simulink model "MRI_2D_FFT"  (R2020a)
settings: Solver=VariableStepAuto  StartTime=0.0  StopTime=256*256*11+2000  RelTol=1e-3  EnableMultiTasking=on
PreLoadFcn:
  | MRI_2D_FFT_PreloadFcn
undefined symbols (not defined in the file): col_in, col_out, corner_turn_memory_depth, row_in, xlFrameDisplay
libraries: xbsIndex_r4 x83, dspswit3 x2, dspsrcs4 x2, xbsCopyrightNotice_r4 x1, simulink x1
settings Model: Creator=dahlawat  LastModifiedBy=viswanad
settings DataIOCC: LimitDataPoints=on  ReturnWorkspaceOutputs=off
settings OptimizationCC: LifeSpan=inf
settings DebuggingCC: AllowSymbolicDim=off  SFUnexpectedBacktrackingDiag=warning  SFNoUnconditionalDefaultTransitionDiag=warning  SFExecutionAtInitializationDiag=none  ArithmeticOperatorsInVariantConditions=warning
settings ModelReferenceCC: PropagateSignalLabelsOutOfModel=off
settings SFSimCC: SimUseLocalCustomCode=off  CustomCodeUndefinedFunction=UseInterfaceOnly
settings RTWCC: RTWUseLocalCustomCode=off
settings CodeAppCC: StateflowObjectComments=on
settings GRTTargetCC: TargetLangStandard=C89/C90 (ANSI)
settings ConfigComp: CovMetricSettings=dw  CovSaveCumulativeToWorkspaceVar=on  CovSaveSingleToWorkspaceVar=on  CovExternalEMLEnable=off

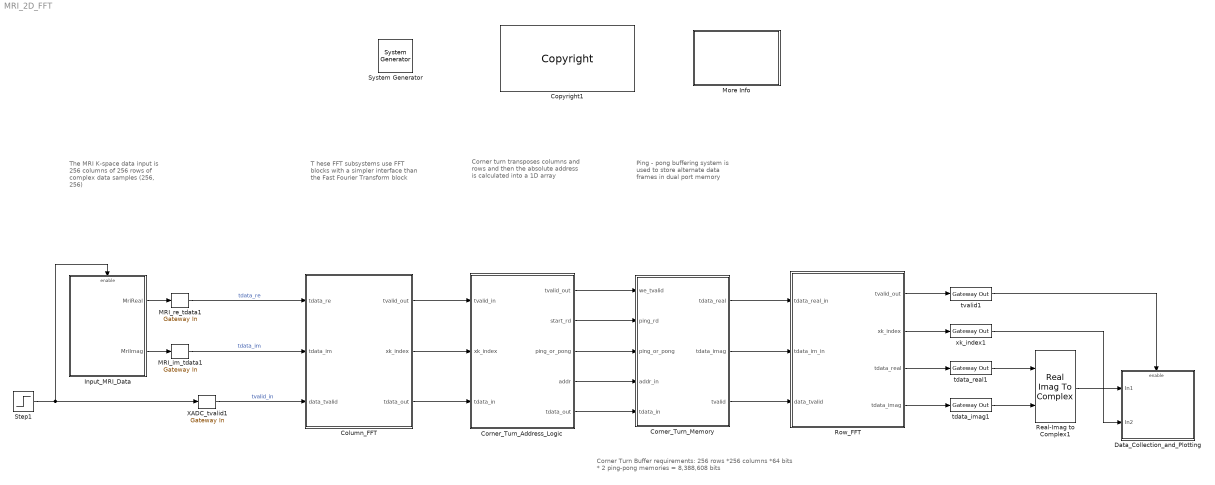
== system MRI_2D_FFT ==
  note: T hese FFT subsystems use FFT blocks with a simpler interface than the Fast Fourier Transform block
  note: Corner Turn Buffer requirements: 256 rows *256 columns *64 bits * 2 ping-pong memories = 8,388,608 bits
  note: The MRI K-space data input is 256 columns of 256 rows of complex data samples
      | (256, 256)
  note: Corner turn transposes columns and rows and then the absolute address is calculated into a 1D array
  note: Ping - pong buffering system is used to store alternate data frames in dual port memory
  " System Generator" : xbsIndex_r4/ System Generator  Tag=genX  xilinxfamily=zynquplus  part=xczu7ev  speed=-2-e  package=ffvc1156  synthesis_tool=Vivado  clock_wrapper=Clock Enables  directory=./netlist  proj_type=Vivado  Synth_file=Vivado Synthesis Defaults  Impl_file=Vivado Implementation Defaults  testbench=on  simulink_period=1  sysclk_period=10  dcm_input_clock_period=10  incr_netlist=off  trim_vbits=Everywhere in SubSystem  dbl_ovrd=According to Block Masks  core_generation=According to Block Masks  run_coregen=off  deprecated_control=off  eval_field=0  block_type=sysgen
  Column_FFT : Subsystem
  Copyright1 : xbsCopyrightNotice_r4/Copyright  copyrighttext="Copyright (c) 2021  by  Xilinx, Inc. All rights reserved.<br><br>This file contains proprietary, confidential information of Xilinx, Inc., is distributed under license from Xilinx, Inc., and may be used, copied and/or disclosed only pursuant to the terms of a valid license agreement with Xilinx, Inc. Xilinx hereby grants you a license to use this file solely for design, simulation, implementation and creation of design files limited to Xilinx devices or technologies. Use with non-Xilinx devices or technologies is expressly prohibited and immediately terminates your license unless covered by a separate agreement.<br><br>Xilinx is providing this design, code, or information \"as-is\" solely for use in developing programs and solutions for Xilinx devices, with no obligation on the part of Xilinx to provide support. By providing this design, code, or information as one possible implementation of this feature, application or standard, Xilinx is making no representation that this implementation is free from any claims of infringement. You are responsible for obtaining any rights you may require for your implementation. Xilinx expressly disclaims any warranty whatsoever with respect to the adequacy of the implementation, including but not limited to any warranties or representations that this implementation is free from claims of infringement, implied warranties of merchantability or fitness for a particular purpose.<br><br>Xilinx products are not intended for use in life support appliances, devices, or systems. Use in such applications is expressly prohibited.<br><br>Any modifications that are made to the Source Code are done at the user's sole risk and will be unsupported.<br><br>This copyright and support notice must be retained as part of this text at all times. (c) Copyright 1995-2021 Xilinx, Inc. All rights reserved."  block_type=copyright
  Corner_Turn_Address_Logic : Subsystem
  Corner_Turn_Memory : Subsystem
  Data_Collection_and_Plotting : Subsystem  TreatAsAtomicUnit=on
  Input_MRI_Data : Subsystem  TreatAsAtomicUnit=on
  MRI_im_tdata1 : xbsIndex_r4/Gateway In  gui_display_data_type=Fixed-point  arith_type=Signed (2's comp)  n_bits=32  bin_pt=31  preci_type=Single  exp_width=8  frac_width=24  rows=1  columns=1  quantization=Truncate  overflow=Wrap  period=1  UseAsADC=off  ADCChannel='1'  interface=None  automatic_assignment=on  address_offset=hex2dec('00')  intf_name=''  intf_description=''  default_value=0  timing_constraint=None  locs_specified=off  LOCs={}  io_standard={}  inherit_from_input=off  hdl_port=on  XmcBlockStatus=1  maskContainerNames=group4  block_type=gatewayin  block_config=sysgen:gateway_in_config
  MRI_re_tdata1 : xbsIndex_r4/Gateway In  gui_display_data_type=Fixed-point  arith_type=Signed (2's comp)  n_bits=32  bin_pt=31  preci_type=Single  exp_width=8  frac_width=24  rows=1  columns=1  quantization=Truncate  overflow=Wrap  period=1  UseAsADC=off  ADCChannel='1'  interface=None  automatic_assignment=on  address_offset=hex2dec('00')  intf_name=''  intf_description=''  default_value=0  timing_constraint=None  locs_specified=off  LOCs={}  io_standard={}  inherit_from_input=off  hdl_port=on  XmcBlockStatus=1  maskContainerNames=group4  block_type=gatewayin  block_config=sysgen:gateway_in_config
  More Info : Subsystem
      mask Display: disp('Double click\n for\n more information.')
  Real-Imag to Complex1 : RealImagToComplex
  Row_FFT : Subsystem
  Step1 : Step  Time=64  SampleTime=1
  XADC_tvalid1 : xbsIndex_r4/Gateway In  gui_display_data_type=Boolean  arith_type=Boolean  n_bits=32  bin_pt=0  preci_type=Single  exp_width=8  frac_width=24  rows=1  columns=1  quantization="Round  (unbiased: +/- Inf)"  overflow=Saturate  period=1  UseAsADC=off  ADCChannel='1'  interface=None  automatic_assignment=on  address_offset=hex2dec('00')  intf_name=''  intf_description=''  default_value=0  timing_constraint=None  locs_specified=off  LOCs={}  io_standard={}  inherit_from_input=off  hdl_port=on  XmcBlockStatus=1  maskContainerNames=group4  block_type=gatewayin  block_config=sysgen:gateway_in_config
  tdata_imag1 : xbsIndex_r4/Gateway Out  inherit_from_input=off  hdl_port=on  rows=1  columns=1  UseAsDAC=off  DACChannel='1'  interface=None  automatic_assignment=on  address_offset=hex2dec('00')  intf_name=''  intf_description=''  timing_constraint=None  locs_specified=off  LOCs={}  io_standard={}  XmcBlockStatus=1  maskContainerNames=group4  block_type=gatewayout  block_config=sysgen:gateway_out_config
  tdata_real1 : xbsIndex_r4/Gateway Out  inherit_from_input=off  hdl_port=on  rows=1  columns=1  UseAsDAC=off  DACChannel='1'  interface=None  automatic_assignment=on  address_offset=hex2dec('00')  intf_name=''  intf_description=''  timing_constraint=None  locs_specified=off  LOCs={}  io_standard={}  XmcBlockStatus=1  maskContainerNames=group4  block_type=gatewayout  block_config=sysgen:gateway_out_config
  tvalid1 : xbsIndex_r4/Gateway Out  inherit_from_input=off  hdl_port=on  rows=1  columns=1  UseAsDAC=off  DACChannel='1'  interface=None  automatic_assignment=on  address_offset=hex2dec('00')  intf_name=''  intf_description=''  timing_constraint=None  locs_specified=off  LOCs={}  io_standard={}  XmcBlockStatus=1  maskContainerNames=group4  block_type=gatewayout  block_config=sysgen:gateway_out_config
  xk_index1 : xbsIndex_r4/Gateway Out  inherit_from_input=off  hdl_port=off  rows=1  columns=1  UseAsDAC=off  DACChannel='1'  interface=None  automatic_assignment=on  address_offset=hex2dec('00')  intf_name=''  intf_description=''  timing_constraint=None  locs_specified=off  LOCs={}  io_standard={}  XmcBlockStatus=1  maskContainerNames=group4  block_type=gatewayout  block_config=sysgen:gateway_out_config
  wires:
  Step1/1 -> Input_MRI_Data/Enable, XADC_tvalid1/1
  XADC_tvalid1/1 -> Column_FFT/3(data_tvalid)  "tvalid_in"
  Input_MRI_Data/1(MriReal) -> MRI_re_tdata1/1
  Input_MRI_Data/2(MriImag) -> MRI_im_tdata1/1
  tvalid1/1 -> Data_Collection_and_Plotting/Enable
  tdata_real1/1 -> Real-Imag to Complex1/1
  tdata_imag1/1 -> Real-Imag to Complex1/2
  Column_FFT/1(tvalid_out) -> Corner_Turn_Address_Logic/1(tvalid_in)
  Column_FFT/2(xk_index) -> Corner_Turn_Address_Logic/2(xk_index)
  Column_FFT/3(tdata_out) -> Corner_Turn_Address_Logic/3(tdata_in)
  Corner_Turn_Address_Logic/1(tvalid_out) -> Corner_Turn_Memory/1(we_tvalid)
  Corner_Turn_Address_Logic/2(start_rd) -> Corner_Turn_Memory/2(ping_rd)
  Corner_Turn_Address_Logic/3(ping_or_pong) -> Corner_Turn_Memory/3(ping_or_pong)
  Corner_Turn_Address_Logic/4(addr) -> Corner_Turn_Memory/4(addr_in)
  Corner_Turn_Address_Logic/5(tdata_out) -> Corner_Turn_Memory/5(tdata_in)
  Corner_Turn_Memory/2(tdata_imag) -> Row_FFT/2(tdata_im_in)
  Corner_Turn_Memory/3(tvalid) -> Row_FFT/3(data_tvalid)
  MRI_re_tdata1/1 -> Column_FFT/1(tdata_re)  "tdata_re"
  MRI_im_tdata1/1 -> Column_FFT/2(tdata_im)  "tdata_im"
  Corner_Turn_Memory/1(tdata_real) -> Row_FFT/1(tdata_real_in)
  Row_FFT/1(tvalid_out) -> tvalid1/1
  Row_FFT/2(xk_index) -> xk_index1/1
  Row_FFT/3(tdata_real) -> tdata_real1/1
  Row_FFT/4(tdata_imag) -> tdata_imag1/1
  xk_index1/1 -> Data_Collection_and_Plotting/2(In2)
  Real-Imag to Complex1/1 -> Data_Collection_and_Plotting/1(In1)

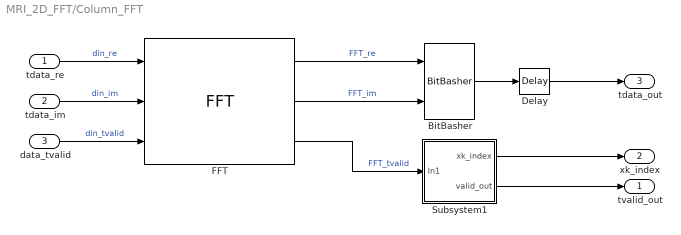
== system MRI_2D_FFT/Column_FFT ==
  tdata_re : Inport
  tdata_im : Inport  Port=2
  data_tvalid : Inport  Port=3
  BitBasher : xbsIndex_r4/BitBasher  bitexpr=a={c,b}  display_expr=off  sr_1=a  arith_type1=Unsigned  bin_pt1=0  sr_2=2  arith_type2=Unsigned  bin_pt2=0  sr_3=3  arith_type3=Unsigned  bin_pt3=0  sr_4=4  arith_type4=Unsigned  bin_pt4=0  XmcBlockStatus=1  maskContainerNames=group1  block_type=bitbasher  block_config=sysgen:BitBasher_config
  Delay : xbsIndex_r4/Delay  rst=off  en=off  latency=1  reg_retiming=off  XmcBlockStatus=1  maskContainerNames=group1  block_type=delay  block_config=sysgen:Delay_config
  FFT : xbsIndex_r4/FFT  transform_length=256  scale_result_by_fft_length=on  bit_reversed_order=on  optimizegoal=Performance  start_frame=on  simulation_type=fast_sim  simulation_model=sysgen:ForwardFFT_Macro  latency=1  XmcBlockStatus=1  maskContainerNames=group1  block_type=xfft_forward  block_config=sysgen:FFTMacro_config
  Subsystem1 : Subsystem
  tvalid_out : Outport  VectorParamsAs1DForOutWhenUnconnected=off
  xk_index : Outport  Port=2  VectorParamsAs1DForOutWhenUnconnected=off
  tdata_out : Outport  Port=3  VectorParamsAs1DForOutWhenUnconnected=off
  wires:
  tdata_im/1 -> FFT/2  "din_im"
  tdata_re/1 -> FFT/1  "din_re"
  data_tvalid/1 -> FFT/3  "din_tvalid"
  BitBasher/1 -> Delay/1
  FFT/3 -> Subsystem1/1(In1)  "FFT_tvalid"
  Subsystem1/2(valid_out) -> tvalid_out/1
  Subsystem1/1(xk_index) -> xk_index/1
  Delay/1 -> tdata_out/1
  FFT/1 -> BitBasher/1  "FFT_re"
  FFT/2 -> BitBasher/2  "FFT_im"

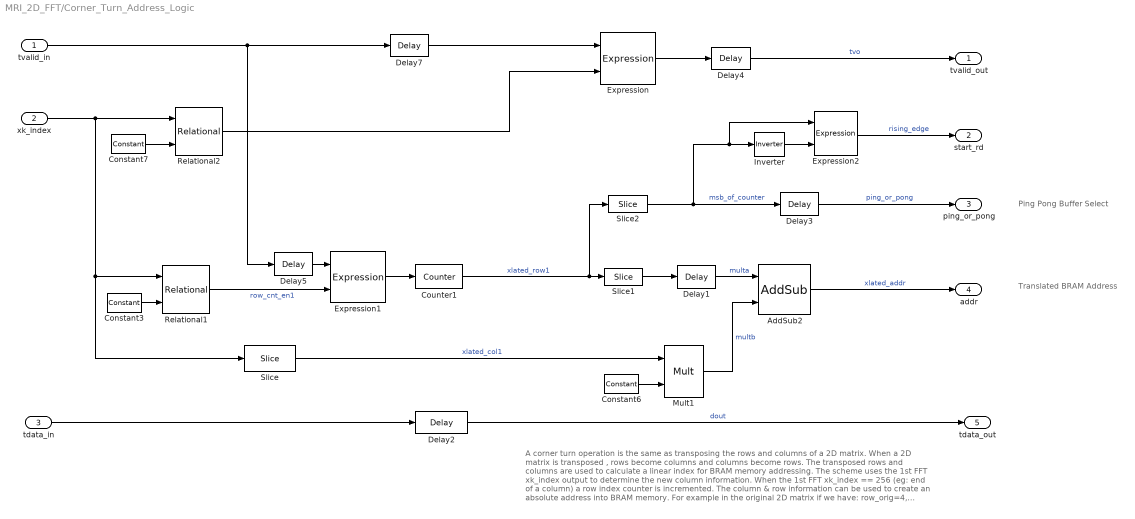
== system MRI_2D_FFT/Corner_Turn_Address_Logic ==
  note: A corner turn operation is the same as transposing the rows and columns of a 2D matrix. When a 2D matrix is transposed , rows become columns and columns become rows. The transposed rows and columns are used to calculate a linear index for BRAM memory addressing.
      |
      | The scheme uses the 1st FFT xk_index output to determine the new column information. When the 1st FFT xk_index == 256 (eg: end of a column) a row index counter is incremented. The column & row information can be used to create an absolute address into BRAM memory.
      |
      | For example in the original 2D matrix if we have: row_orig=4, col_orig=2 (which translates into an absolute address of 4+1*256=260); after transpose the new address is row_new = 2, col_new=4 and therefore the new absolute BRAM address is (col_new) *(length of col - 1) + (row_new) = 3*256+2=770
      |
      | For more info on storing a 2D matrix with a "linear indexing" scheme, please see: http://www.mathworks.com/help/matlab/math/matrix-indexing.html
  note: Ping Pong Buffer Select
  note: Translated BRAM Address
  tvalid_in : Inport
  xk_index : Inport  Port=2
  tdata_in : Inport  Port=3
  AddSub2 : xbsIndex_r4/AddSub  mode=Addition  use_carryin=off  use_carryout=off  en=off  latency=1  precision=User Defined  arith_type=Unsigned  n_bits=log2(col_out*col_in)  bin_pt=0  quantization=Truncate  overflow=Wrap  use_behavioral_HDL=off  hw_selection=Fabric  pipelined=off  XmcBlockStatus=1  maskContainerNames=tabcontainer1  block_type=addsub  block_config=sysgen:Addsub_config
  Constant3 : xbsIndex_r4/Constant  const=col_out-1  gui_display_data_type=Fixed-point  arith_type=Unsigned  n_bits=10  bin_pt=0  preci_type=Single  exp_width=8  frac_width=24  explicit_period=off  period=1  XmcBlockStatus=1  maskContainerNames=tabcontainer1  block_type=constant  block_config=sysgen:Constant_config
  Constant6 : xbsIndex_r4/Constant  const=col_in  gui_display_data_type=Fixed-point  arith_type=Unsigned  n_bits=10  bin_pt=0  preci_type=Single  exp_width=8  frac_width=24  explicit_period=off  period=1  XmcBlockStatus=1  maskContainerNames=tabcontainer1  block_type=constant  block_config=sysgen:Constant_config
  Constant7 : xbsIndex_r4/Constant  const=col_out-1  gui_display_data_type=Fixed-point  arith_type=Unsigned  n_bits=10  bin_pt=0  preci_type=Single  exp_width=8  frac_width=24  explicit_period=off  period=1  XmcBlockStatus=1  maskContainerNames=tabcontainer1  block_type=constant  block_config=sysgen:Constant_config
  Counter1 : xbsIndex_r4/Counter  cnt_type=Free Running  cnt_to=16  operation=Up  start_count=0  cnt_by_val=1  arith_type=Unsigned  n_bits=log2(col_in)+1  bin_pt=0  load_pin=off  rst=off  en=on  explicit_period=on  period=1  use_behavioral_HDL=off  implementation=Fabric  XmcBlockStatus=1  maskContainerNames=group1  block_type=counter  block_config=sysgen:Counter_config
  Delay1 : xbsIndex_r4/Delay  rst=off  en=off  latency=1  reg_retiming=off  XmcBlockStatus=1  maskContainerNames=group1  block_type=delay  block_config=sysgen:Delay_config
  Delay2 : xbsIndex_r4/Delay  rst=off  en=off  latency=4  reg_retiming=off  XmcBlockStatus=1  maskContainerNames=group1  block_type=delay  block_config=sysgen:Delay_config
  Delay3 : xbsIndex_r4/Delay  rst=off  en=off  latency=2  reg_retiming=off  XmcBlockStatus=1  maskContainerNames=group1  block_type=delay  block_config=sysgen:Delay_config
  Delay4 : xbsIndex_r4/Delay  rst=off  en=off  latency=2  reg_retiming=off  XmcBlockStatus=1  maskContainerNames=group1  block_type=delay  block_config=sysgen:Delay_config
  Delay5 : xbsIndex_r4/Delay  rst=off  en=off  latency=1  reg_retiming=off  XmcBlockStatus=1  maskContainerNames=group1  block_type=delay  block_config=sysgen:Delay_config
  Delay7 : xbsIndex_r4/Delay  rst=off  en=off  latency=1  reg_retiming=off  XmcBlockStatus=1  maskContainerNames=group1  block_type=delay  block_config=sysgen:Delay_config
  Expression : xbsIndex_r4/Expression  expression=a & b  align_bp=on  en=off  latency=1  precision=Full  arith_type=Unsigned  n_bits=16  bin_pt=0  XmcBlockStatus=1  maskContainerNames=tabcontainer1  block_type=expr  block_config=sysgen:Expr_config
  Expression1 : xbsIndex_r4/Expression  expression=a & b  align_bp=on  en=off  latency=1  precision=Full  arith_type=Unsigned  n_bits=16  bin_pt=0  XmcBlockStatus=1  maskContainerNames=tabcontainer1  block_type=expr  block_config=sysgen:Expr_config
  Expression2 : xbsIndex_r4/Expression  expression=a & b  align_bp=on  en=off  latency=1  precision=Full  arith_type=Unsigned  n_bits=16  bin_pt=0  XmcBlockStatus=1  maskContainerNames=tabcontainer1  block_type=expr  block_config=sysgen:Expr_config
  Inverter : xbsIndex_r4/Inverter  en=off  latency=1  XmcBlockStatus=1  maskContainerNames=group2  block_type=inv  block_config=sysgen:Inverter_config
  Mult1 : xbsIndex_r4/Mult  precision=Full  arith_type="Signed  (2's comp)"  n_bits=16  bin_pt=14  quantization=Truncate  overflow=Wrap  en=off  latency=3  use_behavioral_HDL=off  opt=Speed  use_embedded=on  optimum_pipeline=off  pipeline=on  use_rpm=on  placement_style=Triangular  XmcBlockStatus=1  maskContainerNames=group1  block_type=mult  block_config=sysgen:Mult_config
  Relational1 : xbsIndex_r4/Relational  mode=a=b  op_type=Bool  en=off  latency=1  XmcBlockStatus=1  maskContainerNames=tabcontainer1  block_type=relational  block_config=sysgen:Relational_config
  Relational2 : xbsIndex_r4/Relational  mode=a<=b  op_type=Bool  en=off  latency=1  XmcBlockStatus=1  maskContainerNames=tabcontainer1  block_type=relational  block_config=sysgen:Relational_config
  Slice : xbsIndex_r4/Slice  nbits=log2(col_out)  boolean_output=off  mode=Lower Bit Location + Width  bit1=0  base1=LSB of Input  bit0=0  base0=LSB of Input  XmcBlockStatus=1  maskContainerNames=group1  block_type=slice  block_config=sysgen:Slice_config
  Slice1 : xbsIndex_r4/Slice  nbits=log2(col_in)  boolean_output=off  mode=Lower Bit Location + Width  bit1=0  base1=LSB of Input  bit0=0  base0=LSB of Input  XmcBlockStatus=1  maskContainerNames=group1  block_type=slice  block_config=sysgen:Slice_config
  Slice2 : xbsIndex_r4/Slice  nbits=1  boolean_output=off  mode=Upper Bit Location + Width  bit1=0  base1=MSB of Input  bit0=0  base0=LSB of Input  XmcBlockStatus=1  maskContainerNames=group1  block_type=slice  block_config=sysgen:Slice_config
  tvalid_out : Outport  VectorParamsAs1DForOutWhenUnconnected=off
  start_rd : Outport  Port=2  VectorParamsAs1DForOutWhenUnconnected=off
  ping_or_pong : Outport  Port=3  VectorParamsAs1DForOutWhenUnconnected=off
  addr : Outport  Port=4  VectorParamsAs1DForOutWhenUnconnected=off
  tdata_out : Outport  Port=5  VectorParamsAs1DForOutWhenUnconnected=off
  wires:
  tdata_in/1 -> Delay2/1
  Delay2/1 -> tdata_out/1  "dout"
  Constant3/1 -> Relational1/2
  Relational1/1 -> Expression1/2  "row_cnt_en1"
  Mult1/1 -> AddSub2/2  "multb"
  Slice/1 -> Mult1/1  "xlated_col1"
  AddSub2/1 -> addr/1  "xlated_addr"
  Constant6/1 -> Mult1/2
  tvalid_in/1 -> Delay7/1, Delay5/1
  Expression/1 -> Delay4/1
  Delay4/1 -> tvalid_out/1  "tvo"
  Counter1/1 -> Slice1/1, Slice2/1  "xlated_row1"
  Delay1/1 -> AddSub2/1  "multa"
  xk_index/1 -> Relational2/1, Relational1/1, Slice/1
  Constant7/1 -> Relational2/2
  Relational2/1 -> Expression/2
  Slice1/1 -> Delay1/1
  Delay3/1 -> ping_or_pong/1  "ping_or_pong"
  Expression1/1 -> Counter1/1
  Delay5/1 -> Expression1/1
  Slice2/1 -> Delay3/1, Expression2/1, Inverter/1  "msb_of_counter"
  Expression2/1 -> start_rd/1  "rising_edge"
  Delay7/1 -> Expression/1
  Inverter/1 -> Expression2/2

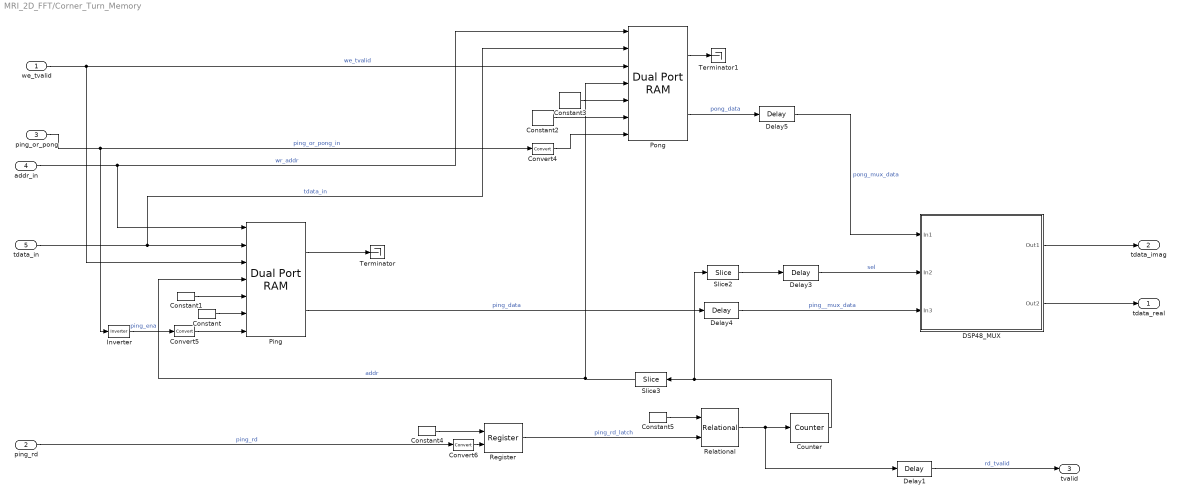
== system MRI_2D_FFT/Corner_Turn_Memory ==
  we_tvalid : Inport
  ping_rd : Inport  Port=2
  ping_or_pong : Inport  Port=3
  addr_in : Inport  Port=4
  tdata_in : Inport  Port=5
  Constant : xbsIndex_r4/Constant  const=0  gui_display_data_type=Boolean  arith_type=Boolean  n_bits=16  bin_pt=14  preci_type=Single  exp_width=8  frac_width=24  explicit_period=off  period=1  XmcBlockStatus=1  maskContainerNames=tabcontainer1  block_type=constant  block_config=sysgen:Constant_config
  Constant1 : xbsIndex_r4/Constant  const=0  gui_display_data_type=Fixed-point  arith_type=Unsigned  n_bits=64  bin_pt=0  preci_type=Single  exp_width=8  frac_width=24  explicit_period=off  period=1  XmcBlockStatus=1  maskContainerNames=tabcontainer1  block_type=constant  block_config=sysgen:Constant_config
  Constant2 : xbsIndex_r4/Constant  const=0  gui_display_data_type=Boolean  arith_type=Boolean  n_bits=16  bin_pt=14  preci_type=Single  exp_width=8  frac_width=24  explicit_period=off  period=1  XmcBlockStatus=1  maskContainerNames=tabcontainer1  block_type=constant  block_config=sysgen:Constant_config
  Constant3 : xbsIndex_r4/Constant  const=0  gui_display_data_type=Fixed-point  arith_type=Unsigned  n_bits=64  bin_pt=0  preci_type=Single  exp_width=8  frac_width=24  explicit_period=off  period=1  XmcBlockStatus=1  maskContainerNames=tabcontainer1  block_type=constant  block_config=sysgen:Constant_config
  Constant4 : xbsIndex_r4/Constant  const=1  gui_display_data_type=Fixed-point  arith_type=Unsigned  n_bits=1  bin_pt=0  preci_type=Single  exp_width=8  frac_width=24  explicit_period=off  period=1  XmcBlockStatus=1  maskContainerNames=tabcontainer1  block_type=constant  block_config=sysgen:Constant_config
  Constant5 : xbsIndex_r4/Constant  const=1  gui_display_data_type=Fixed-point  arith_type=Unsigned  n_bits=1  bin_pt=0  preci_type=Single  exp_width=8  frac_width=24  explicit_period=off  period=1  XmcBlockStatus=1  maskContainerNames=tabcontainer1  block_type=constant  block_config=sysgen:Constant_config
  Convert4 : xbsIndex_r4/Convert  gui_display_data_type=Boolean  arith_type=Boolean  n_bits=16  bin_pt=14  float_type=Single  exp_bits=8  fraction_bits=24  quantization=Truncate  overflow=Wrap  en=off  latency=0  pipeline=off  XmcBlockStatus=1  maskContainerNames=group2  block_type=convert  block_config=sysgen:Convert_config
  Convert5 : xbsIndex_r4/Convert  gui_display_data_type=Boolean  arith_type=Boolean  n_bits=16  bin_pt=14  float_type=Single  exp_bits=8  fraction_bits=24  quantization=Truncate  overflow=Wrap  en=off  latency=0  pipeline=off  XmcBlockStatus=1  maskContainerNames=group2  block_type=convert  block_config=sysgen:Convert_config
  Convert6 : xbsIndex_r4/Convert  gui_display_data_type=Boolean  arith_type=Boolean  n_bits=16  bin_pt=14  float_type=Single  exp_bits=8  fraction_bits=24  quantization=Truncate  overflow=Wrap  en=off  latency=0  pipeline=off  XmcBlockStatus=1  maskContainerNames=group2  block_type=convert  block_config=sysgen:Convert_config
  Counter : xbsIndex_r4/Counter  cnt_type=Free Running  cnt_to=Inf  operation=Up  start_count=0  cnt_by_val=1  arith_type=Unsigned  n_bits=corner_turn_memory_depth+1  bin_pt=0  load_pin=off  rst=off  en=on  explicit_period=on  period=1  use_behavioral_HDL=off  implementation=Fabric  XmcBlockStatus=1  maskContainerNames=group1  block_type=counter  block_config=sysgen:Counter_config
  DSP48_MUX : Subsystem
  Delay1 : xbsIndex_r4/Delay  rst=off  en=off  latency=3  reg_retiming=off  XmcBlockStatus=1  maskContainerNames=group1  block_type=delay  block_config=sysgen:Delay_config
  Delay3 : xbsIndex_r4/Delay  rst=off  en=off  latency=2  reg_retiming=off  XmcBlockStatus=1  maskContainerNames=group1  block_type=delay  block_config=sysgen:Delay_config
  Delay4 : xbsIndex_r4/Delay  rst=off  en=off  latency=1  reg_retiming=off  XmcBlockStatus=1  maskContainerNames=group1  block_type=delay  block_config=sysgen:Delay_config
  Delay5 : xbsIndex_r4/Delay  rst=off  en=off  latency=1  reg_retiming=off  XmcBlockStatus=1  maskContainerNames=group1  block_type=delay  block_config=sysgen:Delay_config
  Inverter : xbsIndex_r4/Inverter  en=off  latency=0  XmcBlockStatus=1  maskContainerNames=group2  block_type=inv  block_config=sysgen:Inverter_config
  Ping : xbsIndex_r4/Dual Port RAM  depth=col_in * col_out  initVector=0  distributed_mem=Ultra RAM  init_a=0  init_b=0  rst_a=off  rst_b=off  en_a=on  en_b=off  latency=1  write_mode_A=No Read On Write  write_mode_B=No Read On Write  optimize=Area  explicit_period=[]  period=[]  simulation_type=fast_sim  XmcBlockStatus=1  maskContainerNames=tabcontainer1  block_type=dpram  block_config=sysgen:Dpram_config
      settings: infoedit=[]
  Pong : xbsIndex_r4/Dual Port RAM  depth=col_in * col_out  initVector=0  distributed_mem=Ultra RAM  init_a=0  init_b=0  rst_a=off  rst_b=off  en_a=on  en_b=off  latency=1  write_mode_A=No Read On Write  write_mode_B=No Read On Write  optimize=Area  explicit_period=[]  period=[]  simulation_type=fast_sim  XmcBlockStatus=1  maskContainerNames=tabcontainer1  block_type=dpram  block_config=sysgen:Dpram_config
      settings: infoedit=[]
  Register : xbsIndex_r4/Register  init=0  rst=off  en=on  XmcBlockStatus=1  maskContainerNames=tabcontainer1  block_type=register  block_config=sysgen:Register_config
  Relational : xbsIndex_r4/Relational  mode=a=b  op_type=Bool  en=off  latency=1  XmcBlockStatus=1  maskContainerNames=tabcontainer1  block_type=relational  block_config=sysgen:Relational_config
  Slice2 : xbsIndex_r4/Slice  nbits=1  boolean_output=off  mode=Upper Bit Location + Width  bit1=0  base1=MSB of Input  bit0=0  base0=LSB of Input  XmcBlockStatus=1  maskContainerNames=group1  block_type=slice  block_config=sysgen:Slice_config
  Slice3 : xbsIndex_r4/Slice  nbits=corner_turn_memory_depth  boolean_output=off  mode=Lower Bit Location + Width  bit1=0  base1=LSB of Input  bit0=0  base0=LSB of Input  XmcBlockStatus=1  maskContainerNames=group1  block_type=slice  block_config=sysgen:Slice_config
  Terminator : Terminator
  Terminator1 : Terminator
  tdata_real : Outport  VectorParamsAs1DForOutWhenUnconnected=off
  tdata_imag : Outport  Port=2  VectorParamsAs1DForOutWhenUnconnected=off
  tvalid : Outport  Port=3  VectorParamsAs1DForOutWhenUnconnected=off
  wires:
  Pong/2 -> Delay5/1  "pong_data"
  Convert4/1 -> Pong/7
  Convert5/1 -> Ping/7
  Pong/1 -> Terminator1/1
  Ping/1 -> Terminator/1
  ping_or_pong/1 -> Convert4/1, Inverter/1  "ping_or_pong_in"
  Inverter/1 -> Convert5/1  "ping_ena"
  addr_in/1 -> Ping/1, Pong/1  "wr_addr"
  tdata_in/1 -> Pong/2, Ping/2  "tdata_in"
  we_tvalid/1 -> Ping/3, Pong/3  "we_tvalid"
  Counter/1 -> Slice2/1, Slice3/1
  Constant/1 -> Ping/6
  Constant1/1 -> Ping/5
  Constant2/1 -> Pong/6
  Constant3/1 -> Pong/5
  Register/1 -> Relational/2  "ping_rd_latch"
  Ping/2 -> Delay4/1  "ping_data"
  Convert6/1 -> Register/2
  Delay1/1 -> tvalid/1  "rd_tvalid"
  Slice2/1 -> Delay3/1
  Slice3/1 -> Ping/4, Pong/4  "addr"
  ping_rd/1 -> Convert6/1  "ping_rd"
  Relational/1 -> Delay1/1, Counter/1
  Constant4/1 -> Register/1
  Constant5/1 -> Relational/1
  Delay5/1 -> DSP48_MUX/1(In1)  "pong_mux_data"
  Delay3/1 -> DSP48_MUX/2(In2)  "sel"
  Delay4/1 -> DSP48_MUX/3(In3)  "ping__mux_data"
  DSP48_MUX/1(Out1) -> tdata_imag/1
  DSP48_MUX/2(Out2) -> tdata_real/1

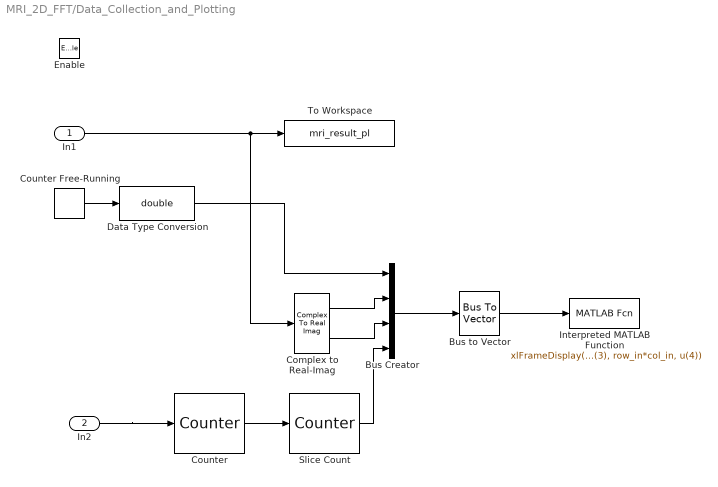
== system MRI_2D_FFT/Data_Collection_and_Plotting ==
  In1 : Inport
  In2 : Inport  Port=2
  Enable : EnablePort
  Bus Creator : BusCreator  Inputs=4
  Bus to Vector : BusToVector
  Complex to Real-Imag : ComplexToRealImag
  Counter : dspswit3/Counter  Direction=Up  CountEvent=Rising edge  CounterSize=User defined  MaxCount=255  InitialCount=0  Output=Count  HitValue=32  ResetInput=off  SamplesPerFrame=1  Ts=1  CntDtype=double  HitDtype=Logical
  Counter Free-Running : simulink/Sources/Counter Free-Running  NumBits=log2(row_in*col_in)  tsamp=1
  Data Type Conversion : DataTypeConversion  OutDataTypeStr=double
  Interpreted MATLAB Function : MATLABFcn  MATLABFcn=xlFrameDisplay(u(1),u(2),u(3), row_in*col_in, u(4))
  Slice Count : dspswit3/Counter  Direction=Up  CountEvent=Rising edge  CounterSize=User defined  MaxCount=10  InitialCount=0  Output=Count  HitValue=32  ResetInput=off  SamplesPerFrame=1  Ts=1  CntDtype=double  HitDtype=Logical
  To Workspace : ToWorkspace  VariableName=mri_result_pl  SampleTime=-1
  wires:
  Counter Free-Running/1 -> Data Type Conversion/1
  Data Type Conversion/1 -> Bus Creator/1
  In1/1 -> Complex to Real-Imag/1, To Workspace/1
  Complex to Real-Imag/1 -> Bus Creator/2
  Complex to Real-Imag/2 -> Bus Creator/3
  Bus Creator/1 -> Bus to Vector/1
  Bus to Vector/1 -> Interpreted MATLAB Function/1
  Slice Count/1 -> Bus Creator/4
  Counter/1 -> Slice Count/1
  In2/1 -> Counter/1

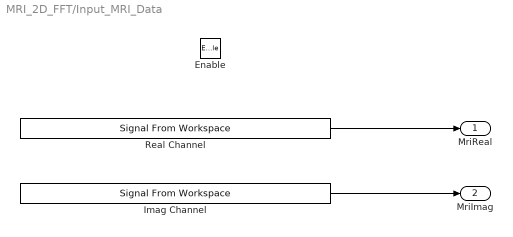
== system MRI_2D_FFT/Input_MRI_Data ==
  Enable : EnablePort
  Imag Channel : dspsrcs4/Signal From Workspace  X=MRIDemo_data_imag_channel  Ts=1  nsamps=1  OutputAfterFinalValue=Setting to zero  ignoreOrWarnInputAndFrameLengths=off  OutputFrames=on
  Real Channel : dspsrcs4/Signal From Workspace  X=MRIDemo_data_real_channel  Ts=1  nsamps=1  OutputAfterFinalValue=Setting to zero  ignoreOrWarnInputAndFrameLengths=off  OutputFrames=on
  MriReal : Outport  VectorParamsAs1DForOutWhenUnconnected=off
  MriImag : Outport  Port=2  VectorParamsAs1DForOutWhenUnconnected=off
  wires:
  Real Channel/1 -> MriReal/1
  Imag Channel/1 -> MriImag/1

== system MRI_2D_FFT/More Info ==
  note: This demo performs a two dimensional FFT (2D-FFT) on input data. Since the FFT is completely separable in two dimensions, a column wise FFT is performed in the input image, followed by row wise FFT to realize the 2D-FFT. An efficient implementation is to transpose the columns and rows in memory using a "corner-turning" technique before performing the 2nd FFT operation. This design performs the transpose before storing the data in memory. A ping-pong memory buffer is used to allow continuous processing on adjacent image frames.
  note: Two dimensional FFT using "Corner-Turning" Matrix Transpose Technique

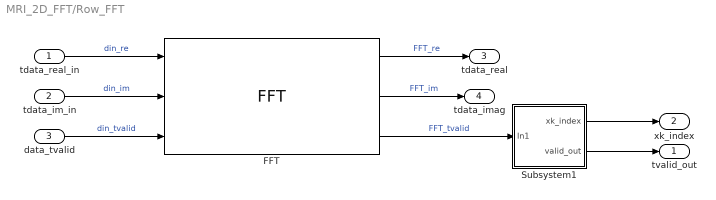
== system MRI_2D_FFT/Row_FFT ==
  tdata_real_in : Inport
  tdata_im_in : Inport  Port=2
  data_tvalid : Inport  Port=3
  FFT : xbsIndex_r4/FFT  transform_length=256  scale_result_by_fft_length=on  bit_reversed_order=on  optimizegoal=Performance  start_frame=on  simulation_type=fast_sim  simulation_model=sysgen:ForwardFFT_Macro  latency=1  XmcBlockStatus=1  maskContainerNames=group1  block_type=xfft_forward  block_config=sysgen:FFTMacro_config
  Subsystem1 : Subsystem
  tvalid_out : Outport  VectorParamsAs1DForOutWhenUnconnected=off
  xk_index : Outport  Port=2  VectorParamsAs1DForOutWhenUnconnected=off
  tdata_real : Outport  Port=3  VectorParamsAs1DForOutWhenUnconnected=off
  tdata_imag : Outport  Port=4  VectorParamsAs1DForOutWhenUnconnected=off
  wires:
  FFT/1 -> tdata_real/1  "FFT_re"
  FFT/3 -> Subsystem1/1(In1)  "FFT_tvalid"
  FFT/2 -> tdata_imag/1  "FFT_im"
  tdata_im_in/1 -> FFT/2  "din_im"
  tdata_real_in/1 -> FFT/1  "din_re"
  data_tvalid/1 -> FFT/3  "din_tvalid"
  Subsystem1/1(xk_index) -> xk_index/1
  Subsystem1/2(valid_out) -> tvalid_out/1

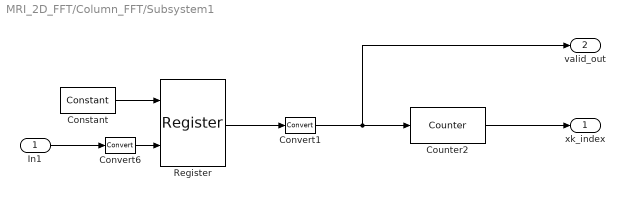
== system MRI_2D_FFT/Column_FFT/Subsystem1 ==
  In1 : Inport
  Constant : xbsIndex_r4/Constant  const=1.0  gui_display_data_type=Fixed-point  arith_type=Unsigned  n_bits=1  bin_pt=0  preci_type=Single  exp_width=8  frac_width=24  explicit_period=on  period=1  XmcBlockStatus=1  maskContainerNames=tabcontainer1  block_type=constant  block_config=sysgen:Constant_config
  Convert1 : xbsIndex_r4/Convert  gui_display_data_type=Boolean  arith_type=Boolean  n_bits=16  bin_pt=14  float_type=Single  exp_bits=8  fraction_bits=24  quantization=Truncate  overflow=Wrap  en=off  latency=0  pipeline=off  XmcBlockStatus=1  maskContainerNames=group2  block_type=convert  block_config=sysgen:Convert_config
  Convert6 : xbsIndex_r4/Convert  gui_display_data_type=Boolean  arith_type=Boolean  n_bits=16  bin_pt=14  float_type=Single  exp_bits=8  fraction_bits=24  quantization=Truncate  overflow=Wrap  en=off  latency=0  pipeline=off  XmcBlockStatus=1  maskContainerNames=group2  block_type=convert  block_config=sysgen:Convert_config
  Counter2 : xbsIndex_r4/Counter  cnt_type=Count Limited  cnt_to=255  operation=Up  start_count=0  cnt_by_val=1  arith_type=Unsigned  n_bits=8  bin_pt=0  load_pin=off  rst=off  en=on  explicit_period=on  period=1  use_behavioral_HDL=off  implementation=Fabric  XmcBlockStatus=1  maskContainerNames=group1  block_type=counter  block_config=sysgen:Counter_config
  Register : xbsIndex_r4/Register  init=0  rst=off  en=on  XmcBlockStatus=1  maskContainerNames=tabcontainer1  block_type=register  block_config=sysgen:Register_config
  xk_index : Outport  VectorParamsAs1DForOutWhenUnconnected=off
  valid_out : Outport  Port=2  VectorParamsAs1DForOutWhenUnconnected=off
  wires:
  In1/1 -> Convert6/1
  Convert6/1 -> Register/2
  Constant/1 -> Register/1
  Register/1 -> Convert1/1
  Convert1/1 -> Counter2/1, valid_out/1
  Counter2/1 -> xk_index/1

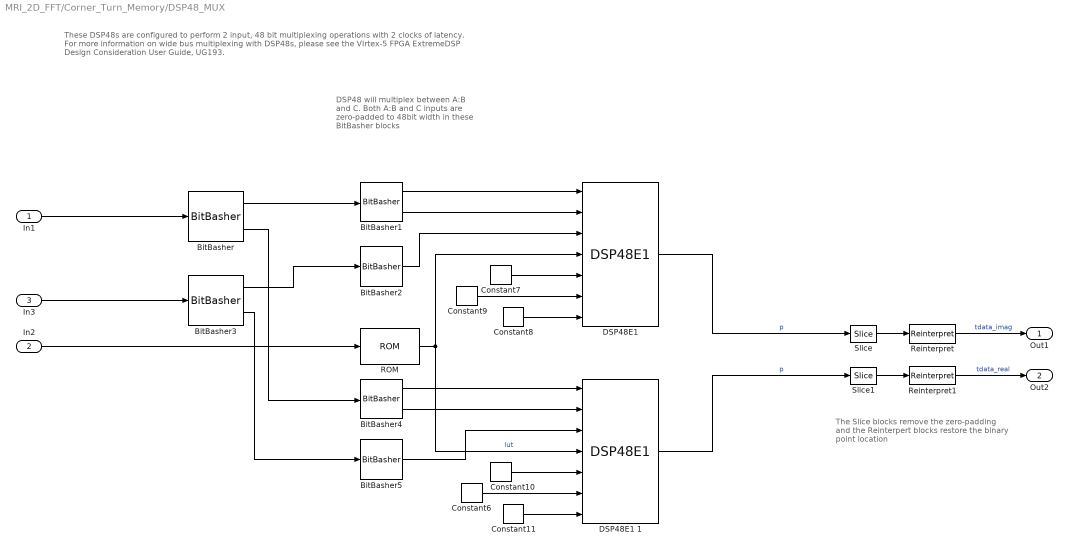
== system MRI_2D_FFT/Corner_Turn_Memory/DSP48_MUX ==
  note: DSP48 will multiplex between A:B and C.
      | Both A:B and C inputs are zero-padded to 48bit width in these BitBasher blocks
  note: These DSP48s are configured to perform 2 input, 48 bit multiplexing operations with 2 clocks of latency.
      | For more information on wide bus multiplexing with DSP48s, please see the
      | VIrtex-5 FPGA ExtremeDSP Design Consideration User Guide, UG193.
  note: The Slice blocks remove the zero-padding and the Reinterpert blocks restore the binary point location
  In1 : Inport
  In2 : Inport  Port=2
  In3 : Inport  Port=3
  BitBasher : xbsIndex_r4/BitBasher  bitexpr=|  display_expr=off  sr_1=imag  arith_type1="Signed  (2's comp)"  bin_pt1=15  sr_2=real  arith_type2="Signed  (2's comp)"  bin_pt2=15  sr_3=3  arith_type3=Unsigned  bin_pt3=0  sr_4=4  arith_type4=Unsigned  bin_pt4=0  XmcBlockStatus=1  maskContainerNames=group1  block_type=bitbasher  block_config=sysgen:BitBasher_config
      | imag={a[63:32]};
      | real = {a[31:0]};
  BitBasher1 : xbsIndex_r4/BitBasher  bitexpr=|  display_expr=off  sr_1=a  arith_type1="Signed  (2's comp)"  bin_pt1=0  sr_2=b  arith_type2="Signed  (2's comp)"  bin_pt2=0  sr_3=3  arith_type3=Unsigned  bin_pt3=0  sr_4=4  arith_type4=Unsigned  bin_pt4=0  XmcBlockStatus=1  maskContainerNames=group1  block_type=bitbasher  block_config=sysgen:BitBasher_config
      | a={16'b0, d[31:18]};
      | b={d[17:0]};
  BitBasher2 : xbsIndex_r4/BitBasher  bitexpr=a={16'b0, b[31:0]};  display_expr=off  sr_1=a  arith_type1="Signed  (2's comp)"  bin_pt1=0  sr_2=b  arith_type2="Signed  (2's comp)"  bin_pt2=0  sr_3=3  arith_type3=Unsigned  bin_pt3=0  sr_4=4  arith_type4=Unsigned  bin_pt4=0  XmcBlockStatus=1  maskContainerNames=group1  block_type=bitbasher  block_config=sysgen:BitBasher_config
  BitBasher3 : xbsIndex_r4/BitBasher  bitexpr=|  display_expr=off  sr_1=imag  arith_type1="Signed  (2's comp)"  bin_pt1=15  sr_2=real  arith_type2="Signed  (2's comp)"  bin_pt2=15  sr_3=3  arith_type3=Unsigned  bin_pt3=0  sr_4=4  arith_type4=Unsigned  bin_pt4=0  XmcBlockStatus=1  maskContainerNames=group1  block_type=bitbasher  block_config=sysgen:BitBasher_config
      | imag={a[63:32]};
      | real = {a[31:0]};
  BitBasher4 : xbsIndex_r4/BitBasher  bitexpr=|  display_expr=off  sr_1=a  arith_type1="Signed  (2's comp)"  bin_pt1=0  sr_2=b  arith_type2="Signed  (2's comp)"  bin_pt2=0  sr_3=3  arith_type3=Unsigned  bin_pt3=0  sr_4=4  arith_type4=Unsigned  bin_pt4=0  XmcBlockStatus=1  maskContainerNames=group1  block_type=bitbasher  block_config=sysgen:BitBasher_config
      | a={16'b0, d[31:18]};
      | b={d[17:0]};
  BitBasher5 : xbsIndex_r4/BitBasher  bitexpr=a={16'b0, b[31:0]};  display_expr=off  sr_1=a  arith_type1="Signed  (2's comp)"  bin_pt1=0  sr_2=b  arith_type2="Signed  (2's comp)"  bin_pt2=0  sr_3=3  arith_type3=Unsigned  bin_pt3=0  sr_4=4  arith_type4=Unsigned  bin_pt4=0  XmcBlockStatus=1  maskContainerNames=group1  block_type=bitbasher  block_config=sysgen:BitBasher_config
  Constant10 : xbsIndex_r4/Constant  const=0  gui_display_data_type=Fixed-point  arith_type=Unsigned  n_bits=4  bin_pt=0  preci_type=Single  exp_width=8  frac_width=24  explicit_period=off  period=1/307.2e6  XmcBlockStatus=1  maskContainerNames=tabcontainer1  block_type=constant  block_config=sysgen:Constant_config
  Constant11 : xbsIndex_r4/Constant  const=0  gui_display_data_type=Fixed-point  arith_type=Unsigned  n_bits=3  bin_pt=0  preci_type=Single  exp_width=8  frac_width=24  explicit_period=off  period=1/307.2e6  XmcBlockStatus=1  maskContainerNames=tabcontainer1  block_type=constant  block_config=sysgen:Constant_config
  Constant6 : xbsIndex_r4/Constant  const=0  gui_display_data_type=Fixed-point  arith_type=Unsigned  n_bits=1  bin_pt=0  preci_type=Single  exp_width=8  frac_width=24  explicit_period=off  period=1/307.2e6  XmcBlockStatus=1  maskContainerNames=tabcontainer1  block_type=constant  block_config=sysgen:Constant_config
  Constant7 : xbsIndex_r4/Constant  const=0  gui_display_data_type=Fixed-point  arith_type=Unsigned  n_bits=4  bin_pt=0  preci_type=Single  exp_width=8  frac_width=24  explicit_period=off  period=1/307.2e6  XmcBlockStatus=1  maskContainerNames=tabcontainer1  block_type=constant  block_config=sysgen:Constant_config
  Constant8 : xbsIndex_r4/Constant  const=0  gui_display_data_type=Fixed-point  arith_type=Unsigned  n_bits=3  bin_pt=0  preci_type=Single  exp_width=8  frac_width=24  explicit_period=off  period=1/307.2e6  XmcBlockStatus=1  maskContainerNames=tabcontainer1  block_type=constant  block_config=sysgen:Constant_config
  Constant9 : xbsIndex_r4/Constant  const=0  gui_display_data_type=Fixed-point  arith_type=Unsigned  n_bits=1  bin_pt=0  preci_type=Single  exp_width=8  frac_width=24  explicit_period=off  period=1/307.2e6  XmcBlockStatus=1  maskContainerNames=tabcontainer1  block_type=constant  block_config=sysgen:Constant_config
  "DSP48E1 " : xbsIndex_r4/DSP48E1   use_a=Direct from A Port  use_b=Direct from B Port  addsub_mode=ONE48  xl_useadderonly=on  xl_dynamicmult=off  enable_preadder=off  reset_preg=off  pattern_from_creg=1  pattern='000000000000'  mask_from_creg=1  pattern_mask='000000000000'  use_op=off  use_creg=on  rst_all=off  en_all=off  use_pcin=off  use_carrycascin=off  use_multsignin=off  use_carryout=off  use_patterndetect=off  use_patternbdetect=off  use_overflow=off  use_underflow=off  use_acout=off  use_bcout=off  use_pcout=off  use_multsignout=off  use_carrycascout=off  pipeline_a=1  pipeline_b=1  pipeline_acout=1  pipeline_bcout=1  pipeline_c=on  pipeline_p=on  pipeline_mult=off  pipeline_opmode=off  pipeline_alumode=off  pipeline_carryin=off  pipeline_carryinsel=off  dreg=off  adreg=off  register_inmode=off  rst_a=off  rst_b=off  rst_c=off  rst_mult=off  rst_p=off  rst_carry_in=off  rst_alumode=off  rst_ctrl=off  reset_port_d=off  reset_port_inmode=off  en_a1=off  en_a2=off  en_b1=off  en_b2=off  en_c=off  en_mult=off  en_p=off  en_carry_in=off  en_alumode=off  en_multcarryin=off  en_ctrl=off  enable_port_regd=off  enable_port_regad=off  enable_port_reginmode=off  use_synth_model=off  simulation_type=fast_sim  XmcBlockStatus=1  maskContainerNames=tabcontainer1  block_type=dsp48e1  block_config=sysgen:DSP48E1_config
  DSP48E1 1 : xbsIndex_r4/DSP48E1   use_a=Direct from A Port  use_b=Direct from B Port  addsub_mode=ONE48  xl_useadderonly=on  xl_dynamicmult=off  enable_preadder=off  reset_preg=off  pattern_from_creg=1  pattern='000000000000'  mask_from_creg=1  pattern_mask='000000000000'  use_op=off  use_creg=on  rst_all=off  en_all=off  use_pcin=off  use_carrycascin=off  use_multsignin=off  use_carryout=off  use_patterndetect=off  use_patternbdetect=off  use_overflow=off  use_underflow=off  use_acout=off  use_bcout=off  use_pcout=off  use_multsignout=off  use_carrycascout=off  pipeline_a=1  pipeline_b=1  pipeline_acout=1  pipeline_bcout=1  pipeline_c=on  pipeline_p=on  pipeline_mult=off  pipeline_opmode=off  pipeline_alumode=off  pipeline_carryin=off  pipeline_carryinsel=off  dreg=off  adreg=off  register_inmode=off  rst_a=off  rst_b=off  rst_c=off  rst_mult=off  rst_p=off  rst_carry_in=off  rst_alumode=off  rst_ctrl=off  reset_port_d=off  reset_port_inmode=off  en_a1=off  en_a2=off  en_b1=off  en_b2=off  en_c=off  en_mult=off  en_p=off  en_carry_in=off  en_alumode=off  en_multcarryin=off  en_ctrl=off  enable_port_regd=off  enable_port_regad=off  enable_port_reginmode=off  use_synth_model=off  simulation_type=fast_sim  XmcBlockStatus=1  maskContainerNames=tabcontainer1  block_type=dsp48e1  block_config=sysgen:DSP48E1_config
  ROM : xbsIndex_r4/ROM  depth=2  initVector={12, 03}  distributed_mem=Distributed memory  rst=off  init_reg=0  en=off  latency=0  optimize_latency=off  gui_display_data_type=Fixed-point  arith_type=Unsigned  n_bits=7  bin_pt=0  preci_type=Single  exp_width=8  frac_width=24  optimize=Speed  use_rpm=on  simulation_type=fast_sim  XmcBlockStatus=1  maskContainerNames=tabcontainer1  block_type=sprom  block_config=sysgen:SPROM_config
  Reinterpret : xbsIndex_r4/Reinterpret  force_arith_type=on  arith_type="Signed  (2's comp)"  force_bin_pt=on  bin_pt=31  XmcBlockStatus=1  maskContainerNames=group1  block_type=reinterpret  block_config=sysgen:Reinterpret_config
  Reinterpret1 : xbsIndex_r4/Reinterpret  force_arith_type=on  arith_type="Signed  (2's comp)"  force_bin_pt=on  bin_pt=31  XmcBlockStatus=1  maskContainerNames=group1  block_type=reinterpret  block_config=sysgen:Reinterpret_config
  Slice : xbsIndex_r4/Slice  nbits=32  boolean_output=off  mode=Lower Bit Location + Width  bit1=0  base1=MSB of Input  bit0=0  base0=LSB of Input  XmcBlockStatus=1  maskContainerNames=group1  block_type=slice  block_config=sysgen:Slice_config
  Slice1 : xbsIndex_r4/Slice  nbits=32  boolean_output=off  mode=Lower Bit Location + Width  bit1=0  base1=MSB of Input  bit0=0  base0=LSB of Input  XmcBlockStatus=1  maskContainerNames=group1  block_type=slice  block_config=sysgen:Slice_config
  Out1 : Outport  VectorParamsAs1DForOutWhenUnconnected=off
  Out2 : Outport  Port=2  VectorParamsAs1DForOutWhenUnconnected=off
  wires:
  Constant9/1 -> "DSP48E1 "/6
  BitBasher1/1 -> "DSP48E1 "/1
  BitBasher1/2 -> "DSP48E1 "/2
  ROM/1 -> "DSP48E1 "/4, DSP48E1 1/4  "lut"
  Constant7/1 -> "DSP48E1 "/5
  Constant8/1 -> "DSP48E1 "/7
  "DSP48E1 "/1 -> Slice/1  "p"
  BitBasher2/1 -> "DSP48E1 "/3
  BitBasher/1 -> BitBasher1/1
  BitBasher3/1 -> BitBasher2/1
  Constant6/1 -> DSP48E1 1/6
  BitBasher4/1 -> DSP48E1 1/1
  BitBasher4/2 -> DSP48E1 1/2
  Constant10/1 -> DSP48E1 1/5
  Constant11/1 -> DSP48E1 1/7
  BitBasher5/1 -> DSP48E1 1/3
  DSP48E1 1/1 -> Slice1/1  "p"
  BitBasher/2 -> BitBasher4/1
  BitBasher3/2 -> BitBasher5/1
  Reinterpret/1 -> Out1/1  "tdata_imag"
  Reinterpret1/1 -> Out2/1  "tdata_real"
  Slice/1 -> Reinterpret/1
  Slice1/1 -> Reinterpret1/1
  In2/1 -> ROM/1
  In3/1 -> BitBasher3/1
  In1/1 -> BitBasher/1

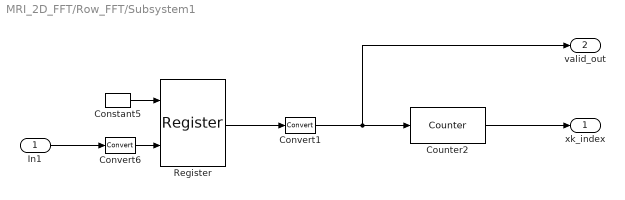
== system MRI_2D_FFT/Row_FFT/Subsystem1 ==
  In1 : Inport
  Constant5 : xbsIndex_r4/Constant  const=1  gui_display_data_type=Fixed-point  arith_type=Unsigned  n_bits=1  bin_pt=0  preci_type=Single  exp_width=8  frac_width=24  explicit_period=off  period=1  XmcBlockStatus=1  maskContainerNames=tabcontainer1  block_type=constant  block_config=sysgen:Constant_config
  Convert1 : xbsIndex_r4/Convert  gui_display_data_type=Boolean  arith_type=Boolean  n_bits=16  bin_pt=14  float_type=Single  exp_bits=8  fraction_bits=24  quantization=Truncate  overflow=Wrap  en=off  latency=0  pipeline=off  XmcBlockStatus=1  maskContainerNames=group2  block_type=convert  block_config=sysgen:Convert_config
  Convert6 : xbsIndex_r4/Convert  gui_display_data_type=Boolean  arith_type=Boolean  n_bits=16  bin_pt=14  float_type=Single  exp_bits=8  fraction_bits=24  quantization=Truncate  overflow=Wrap  en=off  latency=0  pipeline=off  XmcBlockStatus=1  maskContainerNames=group2  block_type=convert  block_config=sysgen:Convert_config
  Counter2 : xbsIndex_r4/Counter  cnt_type=Count Limited  cnt_to=255  operation=Up  start_count=0  cnt_by_val=1  arith_type=Unsigned  n_bits=8  bin_pt=0  load_pin=off  rst=off  en=on  explicit_period=on  period=1  use_behavioral_HDL=off  implementation=Fabric  XmcBlockStatus=1  maskContainerNames=group1  block_type=counter  block_config=sysgen:Counter_config
  Register : xbsIndex_r4/Register  init=0  rst=off  en=on  XmcBlockStatus=1  maskContainerNames=tabcontainer1  block_type=register  block_config=sysgen:Register_config
  xk_index : Outport  VectorParamsAs1DForOutWhenUnconnected=off
  valid_out : Outport  Port=2  VectorParamsAs1DForOutWhenUnconnected=off
  wires:
  In1/1 -> Convert6/1
  Convert6/1 -> Register/2
  Constant5/1 -> Register/1
  Register/1 -> Convert1/1
  Convert1/1 -> Counter2/1, valid_out/1
  Counter2/1 -> xk_index/1
